simulink model "model"  (R2016a)
settings: Solver=VariableStepAuto  SolverMode=SingleTasking  StartTime=0.0  StopTime=10  RelTol=1e-3
InitFcn:
  | data;
  | ControllerVariant = 'RL';
  | load('rlAgent.mat');
  | doTraining = false;
undefined symbols (not defined in the file): dataType, DiscIntNeverNeededParam, inverter, PI_params, pmsm, PU_System, sigbuilder_block, target, Ts, Ts_motor, Ts_simulink, Ts_speed
libraries: mcbcontrolslib x18, mcbpositiondecoderlib x6, simulink x2, mcbplantlib x1, rllib x1, autolibpmsmexterior x1
settings Model: Creator=Muhammad Umer  LastModifiedBy=Zonularity
settings DataIOCC: ReturnWorkspaceOutputs=on
settings DebuggingCC: ParameterPrecisionLossMsg=none  SFUnexpectedBacktrackingDiag=error  SFNoUnconditionalDefaultTransitionDiag=error
settings SFSimCC: SimUseLocalCustomCode=on
settings RTWCC: RTWUseLocalCustomCode=on
settings GRTTargetCC: TargetLangStandard=C99 (ISO)
settings ConfigComp: CovMetricSettings=dwe  CovSaveCumulativeToWorkspaceVar=off  CovSaveSingleToWorkspaceVar=off  CovExternalEMLEnable=on

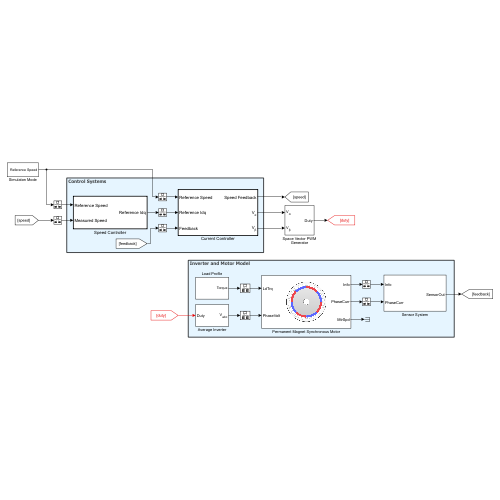
[thumbnail: Simulink's stored preview of the top-level diagram]
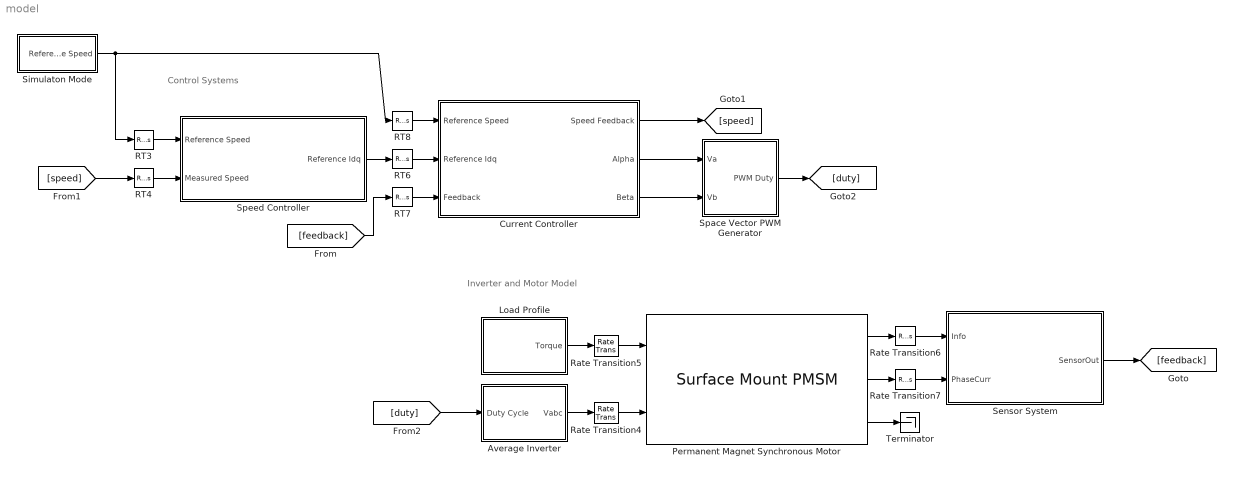
== system model ==
  note: Control Systems
  note: Inverter and Motor Model
  Average Inverter : Subsystem
      mask Display:
      | port_label('input', 1, 'Duty', 'texmode', 'on');
      | port_label('output', 1, 'V_{abc}', 'texmode', 'on');
  Current Controller : Subsystem  TreatAsAtomicUnit=on  mask(Current Controller){contType=PI Controller}
      mask prompts: contType "Controller Type"
      mask help:
      | This block implements the current control loop to generate the desired duty cycle.
      |
      | Choose between a conventional PI Controller and an optimized TD3 Agent.
      mask init:
      | selector = get_param(gcb,'contType');
      | 
      | variantSubsystem = [gcb, '/Control Variant Subsystem']; 
      | 
      | if strcmp(selector,'TD3 Agent')
      |     set_param(variantSubsystem, 'LabelModeActiveChoice', 'RL');
      | else
      |     set_param(variantSubsystem, 'LabelModeActiveChoice', 'PI');
      | end
      settings: OpenFcn=open_system(gcb,'mask');
      mask TypeOptions contType: TD3 Agent | PI Controller
      mask Display:
      | port_label('input', 1, 'Reference Speed', 'texmode', 'on');
      | port_label('input', 2, 'Reference Idq', 'texmode', 'on');
      | port_label('input', 3, 'Feedback', 'texmode', 'on');
      | port_label('output', 1, 'Speed Feedback', 'texmode', 'on');
      | port_label('output', 2, 'V_{\alpha}', 'texmode', 'on');
      | port_label('output', 3, 'V_{\beta}', 'texmode', 'on');
  Load Profile : Subsystem
  Permanent Magnet Synchronous Motor : autolibpmsmexterior/Surface Mount PMSM  port_config=Torque  sim_type=Discrete  Ts=Ts_motor  P=pmsm.p  Rs=pmsm.Rs  Ldq_=pmsm.Ld  KConstText=Permanent flux linkage constant (lambda_pm):  lambda_pm=pmsm.FluxPM  Ke=159.9771  Kt=1.323  mechanical=[pmsm.J, pmsm.B*0, 0]  idq0=[0 0]  theta_init=0  omega_init=0  KConst=pmsm.FluxPM  lambda_pm_calc=pmsm.FluxPM  RefBlkName='autolibpmsmexterior/Surface Mount PMSM'  aMode=5  Ldq="[0.0002      0.0002]"
  RT3 : RateTransition  Deterministic=off  OutPortSampleTime=Ts_speed
  RT4 : RateTransition  Deterministic=off  OutPortSampleTime=Ts_speed
  RT6 : RateTransition  Deterministic=off  OutPortSampleTime=Ts
  RT7 : RateTransition  Deterministic=off  OutPortSampleTime=Ts
  RT8 : RateTransition  Deterministic=off  OutPortSampleTime=Ts
  Rate Transition4 : RateTransition  Deterministic=off  OutPortSampleTime=Ts_motor
  Rate Transition5 : RateTransition  Deterministic=off  OutPortSampleTime=Ts_motor
  Rate Transition6 : RateTransition  Deterministic=off  OutPortSampleTime=Ts_simulink
  Rate Transition7 : RateTransition  Deterministic=off  OutPortSampleTime=Ts_simulink
  Sensor System : Subsystem
      mask Display:
      | port_label('input', 1, 'Info', 'texmode', 'on');
      | port_label('input', 2, 'PhaseCurr', 'texmode', 'on');
      | port_label('output', 1, 'SensorOut', 'texmode', 'on');
  Simulaton Mode : Subsystem  mask(Simulation Mode){Mode=Simulate}
      mask help:
      | Choose simulation mode.
      |
      | Use the training script if the mode is selected to 'Train' Simply run otherwise.
      mask init:
      | selector = get_param(gcb,'Mode');
      | 
      | variantSubsystem = [gcb, '/SimMode']; 
      | 
      | if strcmp(selector,'Simulate')
      |     set_param(variantSubsystem, 'LabelModeActiveChoice', 'simulate');
      | else
      |     set_param(variantSubsystem, 'LabelModeActiveChoice', 'train');
      | end
      settings: OpenFcn=open_system(gcb,'mask');
      mask TypeOptions Mode: Simulate | Train
  Space Vector PWM Generator : Subsystem
      mask Display:
      | color('black');
      | port_label('input', 1, 'V_{\alpha}', 'texmode', 'on');
      | port_label('input', 2, 'V_{\beta}', 'texmode', 'on');
      | port_label('output', 1, 'Duty', 'texmode', 'on');
  Speed Controller : Subsystem  TreatAsAtomicUnit=on  SystemSampleTime=Ts_speed
      mask Display:
      | port_label('input', 1, 'Reference Speed', 'texmode', 'on');
      | port_label('input', 2, 'Measured Speed', 'texmode', 'on');
      | port_label('output', 1, 'Reference Idq', 'texmode', 'on');
  Terminator : Terminator
  wires:
  Rate Transition6/1 -> Sensor System/1(Info)
  Rate Transition4/1 -> Permanent Magnet Synchronous Motor/2
  Rate Transition7/1 -> Sensor System/2(PhaseCurr)
  Load Profile/1(Torque) -> Rate Transition5/1
  Permanent Magnet Synchronous Motor/2 -> Rate Transition7/1
  Average Inverter/1(Vabc) -> Rate Transition4/1
  [speed] -> RT4/1
  Speed Controller/1(Reference Idq) -> RT6/1
  Rate Transition5/1 -> Permanent Magnet Synchronous Motor/1
  Permanent Magnet Synchronous Motor/1 -> Rate Transition6/1
  [feedback] -> RT7/1
  Sensor System/1(SensorOut) -> [feedback]
  Permanent Magnet Synchronous Motor/3 -> Terminator/1
  RT3/1 -> Speed Controller/1(Reference Speed)
  RT4/1 -> Speed Controller/2(Measured Speed)
  [duty] -> Average Inverter/1(Duty Cycle)
  RT8/1 -> Current Controller/1(Reference Speed)
  RT6/1 -> Current Controller/2(Reference Idq)
  RT7/1 -> Current Controller/3(Feedback)
  Current Controller/1(Speed Feedback) -> [speed]
  Simulaton Mode/1(Reference Speed) -> RT3/1, RT8/1
  Current Controller/2(Alpha) -> Space Vector PWM Generator/1(Va)
  Current Controller/3(Beta) -> Space Vector PWM Generator/2(Vb)
  Space Vector PWM Generator/1(PWM Duty) -> [duty]

== system model/Average Inverter ==
  Duty Cycle : Inport
  Average-Value Inverter : mcbplantlib/Average-Value Inverter
  Constant2 : Constant  Value=inverter.V_dc  OutDataTypeStr=single  SampleTime=-1
  Data Type Conversion1 : DataTypeConversion  OutDataTypeStr=single  RndMeth=Simplest
  Rate Transition3 : RateTransition  Integrity=off  Deterministic=off  OutPortSampleTime=Ts_inverter
  Vabc : Outport
  wires:
  Constant2/1 -> Average-Value Inverter/2
  Data Type Conversion1/1 -> Rate Transition3/1
  Rate Transition3/1 -> Average-Value Inverter/1
  Duty Cycle/1 -> Data Type Conversion1/1
  Average-Value Inverter/1 -> Vabc/1

== system model/Current Controller ==
  Reference Speed : Inport
  Reference Idq : Inport  Port=2
  Feedback : Inport  Port=3
  Control Variant Subsystem : Subsystem  Variant=on  OverrideUsingVariant=PI
  Speed Feedback : Outport
  Alpha : Outport  Port=2
  Beta : Outport  Port=3
  wires:
  Control Variant Subsystem/2(Alpha) -> Alpha/1
  Control Variant Subsystem/3(Beta) -> Beta/1
  Control Variant Subsystem/1(Speed Feedback) -> Speed Feedback/1
  Reference Speed/1 -> Control Variant Subsystem/1(Reference Speed)
  Reference Idq/1 -> Control Variant Subsystem/2(Reference Idq)
  Feedback/1 -> Control Variant Subsystem/3(Feedback)

== system model/Load Profile ==
  Data Type Conversion : DataTypeConversion  OutDataTypeStr=single
  Final load : Constant  Value=0.8 * pmsm.T_rated
  IIR Filter : mcbcontrolslib/IIR Filter  VariantControl=Low Pass Filter  VariantSelect=Low-pass  Filter_constant=0.001  advancedSettings=off  Ts=50e-6  cutOff_freq=3.1863
  Motor load : Constant  Commented=on  Value=pmsm.B*pmsm.N_base*2*pi/60
  Switch : Switch  Criteria=u2 > Threshold
  Torque change : Step  Time=19.5  SampleTime=Ts_simulink
  Torque load : Step  Before=0.05*pmsm.T_rated  After=0.5*pmsm.T_rated  SampleTime=Ts_simulink
  Torque : Outport
  wires:
  Switch/1 -> Data Type Conversion/1
  Data Type Conversion/1 -> IIR Filter/1
  Torque change/1 -> Switch/2
  Torque load/1 -> Switch/3
  Final load/1 -> Switch/1
  IIR Filter/1 -> Torque/1

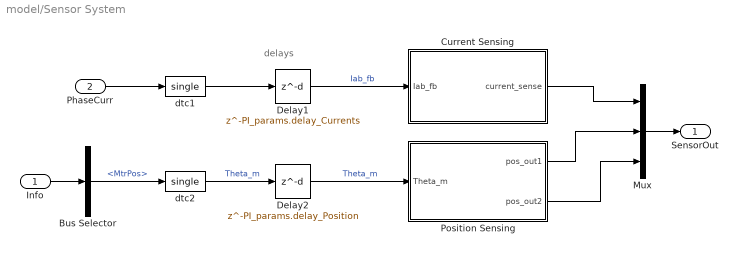
== system model/Sensor System ==
  note: delays
  Info : Inport
  PhaseCurr : Inport  Port=2
  Bus Selector : BusSelector  OutputSignals=MtrPos
  Current Sensing : Subsystem
  Delay1 : Delay  DelayLength=PI_params.delay_Currents
  Delay2 : Delay  DelayLength=PI_params.delay_Position
  Mux : Mux  Inputs=3
  Position Sensing : Subsystem
  dtc1 : DataTypeConversion  OutDataTypeStr=single  RndMeth=Simplest
  dtc2 : DataTypeConversion  OutDataTypeStr=single  RndMeth=Simplest
  SensorOut : Outport
  wires:
  Info/1 -> Bus Selector/1
  PhaseCurr/1 -> dtc1/1
  Bus Selector/1 -> dtc2/1  "<MtrPos>"
  dtc2/1 -> Delay2/1  "Theta_m"
  dtc1/1 -> Delay1/1
  Delay2/1 -> Position Sensing/1(Theta_m)  "Theta_m"
  Delay1/1 -> Current Sensing/1(Iab_fb)  "Iab_fb"
  Current Sensing/1(current_sense) -> Mux/1
  Position Sensing/1(pos_out1) -> Mux/2
  Position Sensing/2(pos_out2) -> Mux/3
  Mux/1 -> SensorOut/1

== system model/Simulaton Mode ==
  SimMode : Subsystem  Variant=on  OverrideUsingVariant=simulate
  Reference Speed : Outport
  wires:
  SimMode/1(Reference Speed) -> Reference Speed/1

== system model/Space Vector PWM Generator ==
  Va : Inport
  Vb : Inport  Port=2
  Mux : Mux  Inputs=3
  Output Scaling : Subsystem
      mask Display:
      | port_label('input', 1, 'V_{abc}', 'texmode', 'on');
      | port_label('output', 1, 'Duty', 'texmode', 'on');
  Space Vector Generator : mcbcontrolslib/Space Vector Generator  inSignal=Valphabeta  modType=SVM: space vector modulation
      link override Modulation method: LabelModeActiveChoice=SVM: space vector modulation
      link override Voltage Input: LabelModeActiveChoice=Valphabeta
  PWM Duty : Outport
  wires:
  Va/1 -> Space Vector Generator/1
  Mux/1 -> Output Scaling/1(Vabc)
  Space Vector Generator/1 -> Mux/1
  Space Vector Generator/3 -> Mux/3
  Space Vector Generator/2 -> Mux/2
  Output Scaling/1(PWM Duty) -> PWM Duty/1
  Vb/1 -> Space Vector Generator/2

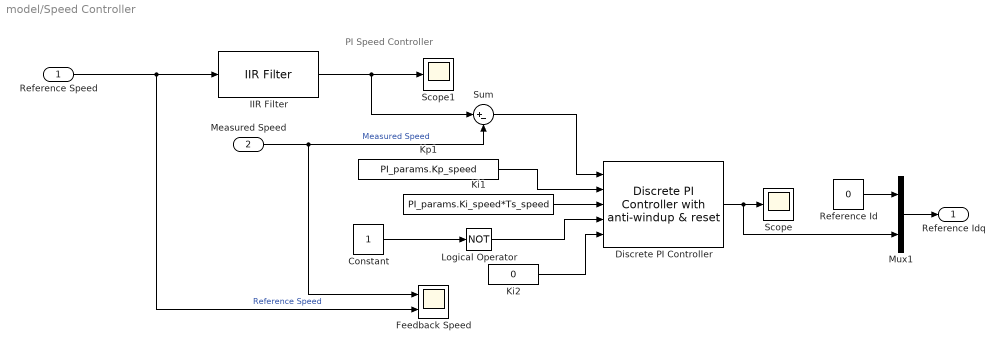
== system model/Speed Controller ==
  note: PI Speed Controller
  Reference Speed : Inport
  Measured Speed : Inport  Port=2
  Constant : Constant  OutDataTypeStr=boolean
  Discrete PI Controller : mcbcontrolslib/Discrete PI Controller  with anti-windup & reset  Controller=PI  UpperSaturationLimit=1  LowerSaturationLimit=-1  IntegratorRTWStateStorageClass=Auto  FilterRTWStateStorageClass=Auto
  Feedback Speed : Scope  NumInputPorts=2
  IIR Filter : mcbcontrolslib/IIR Filter  VariantControl=Low Pass Filter  VariantSelect=Low-pass  Filter_constant=0.01*(Ts_speed/Ts)  advancedSettings=off  Ts=50e-6  cutOff_freq=353.6777
  Ki1 : Constant  Value=PI_params.Ki_speed*Ts_speed  OutDataTypeStr=dataType  SampleTime=-1
  Ki2 : Constant  Value=0  OutDataTypeStr=dataType  SampleTime=-1
  Kp1 : Constant  Value=PI_params.Kp_speed  OutDataTypeStr=dataType  SampleTime=-1
  Logical Operator : Logic  Operator=NOT  IconShape=distinctive  AllPortsSameDT=off  OutDataTypeStr=boolean
  Mux1 : Mux  Inputs=2
  Reference Id : Constant  Value=0  OutDataTypeStr=dataType  SampleTime=Ts_speed
  Scope : Scope
  Scope1 : Scope
  Sum : Sum  Inputs=|+-  OutDataTypeStr=Inherit: Same as first input
  Reference Idq : Outport
  wires:
  Measured Speed/1 -> Feedback Speed/1, Sum/2  "Measured Speed"
  Reference Speed/1 -> Feedback Speed/2, IIR Filter/1  "Reference Speed"
  Reference Id/1 -> Mux1/1
  Mux1/1 -> Reference Idq/1
  IIR Filter/1 -> Sum/1, Scope1/1
  Sum/1 -> Discrete PI Controller/1
  Kp1/1 -> Discrete PI Controller/2
  Ki1/1 -> Discrete PI Controller/3
  Logical Operator/1 -> Discrete PI Controller/4
  Ki2/1 -> Discrete PI Controller/5
  Discrete PI Controller/1 -> Mux1/2, Scope/1
  Constant/1 -> Logical Operator/1

== system model/Current Controller/Control Variant Subsystem ==
  Reference Speed : Inport
  Reference Idq : Inport  Port=2
  Feedback : Inport  Port=3
  PI Controller : Subsystem  VariantControl=PI
  TD3 Agent : Subsystem  VariantControl=RL
  Speed Feedback : Outport
  Alpha : Outport  Port=2
  Beta : Outport  Port=3

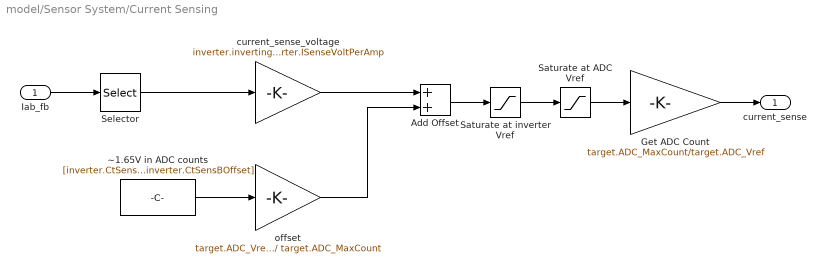
== system model/Sensor System/Current Sensing ==
  Iab_fb : Inport
  Add Offset : Sum  RndMeth=Simplest
  Get ADC Count : Gain  Gain=target.ADC_MaxCount/target.ADC_Vref  OutMin=0  OutMax=target.ADC_MaxCount  OutDataTypeStr=uint16  RndMeth=Simplest
  Saturate at ADC Vref : Saturate  UpperLimit=target.ADC_Vref  LowerLimit=0
  Saturate at inverter Vref : Saturate  UpperLimit=inverter.ISenseVref  LowerLimit=0
  Selector : Selector  InputPortWidth=3  IndexOptions=Index vector (dialog)  Indices=[1 2]  OutputSizes=1
  current_sense_voltage : Gain  Gain=inverter.invertingAmp * inverter.ISenseVoltPerAmp  RndMeth=Simplest  OutDataTypeStr=Inherit: Same as input
  offset : Gain  Gain=target.ADC_Vref / target.ADC_MaxCount  RndMeth=Simplest
  ~1.65V in ADC counts : Constant  Value=[inverter.CtSensAOffset inverter.CtSensBOffset]  OutDataTypeStr=uint16  SampleTime=-1
  current_sense : Outport
  wires:
  Iab_fb/1 -> Selector/1
  current_sense_voltage/1 -> Add Offset/1
  Get ADC Count/1 -> current_sense/1
  ~1.65V in ADC counts/1 -> offset/1
  offset/1 -> Add Offset/2
  Saturate at ADC Vref/1 -> Get ADC Count/1
  Selector/1 -> current_sense_voltage/1
  Saturate at inverter Vref/1 -> Saturate at ADC Vref/1
  Add Offset/1 -> Saturate at inverter Vref/1

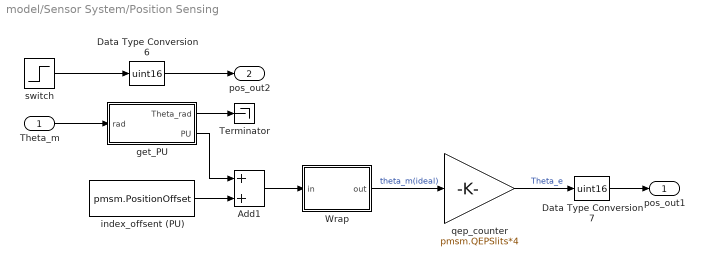
== system model/Sensor System/Position Sensing ==
  Theta_m : Inport
  Add1 : Sum  RndMeth=Simplest
  Data Type Conversion6 : DataTypeConversion  OutDataTypeStr=uint16  RndMeth=Simplest
  Data Type Conversion7 : DataTypeConversion  OutDataTypeStr=uint16  RndMeth=Simplest
  Terminator : Terminator
  Wrap : Subsystem
  "get_PU " : Subsystem
  index_offsent (PU) : Constant  Value=pmsm.PositionOffset  OutDataTypeStr=single  SampleTime=-1
  qep_counter : Gain  Gain=pmsm.QEPSlits*4  OutDataTypeStr=uint16  RndMeth=Simplest
  switch : Step  Time=0.1  SampleTime=Ts_motor
  pos_out1 : Outport
  pos_out2 : Outport  Port=2
  wires:
  Add1/1 -> Wrap/1(in)
  index_offsent (PU)/1 -> Add1/2
  qep_counter/1 -> Data Type Conversion7/1  "Theta_e"
  Theta_m/1 -> "get_PU "/1(rad)
  Data Type Conversion7/1 -> pos_out1/1
  Data Type Conversion6/1 -> pos_out2/1
  switch/1 -> Data Type Conversion6/1
  Wrap/1(out) -> qep_counter/1  "theta_m(ideal)"
  "get_PU "/2(PU) -> Add1/1
  "get_PU "/1(Theta_rad) -> Terminator/1

== system model/Simulaton Mode/SimMode ==
  Simulator : Subsystem  VariantControl=simulate
  Trainer : Subsystem  VariantControl=train
  Reference Speed : Outport

== system model/Space Vector PWM Generator/Output Scaling ==
  Vabc : Inport
  Constant : Constant  Value=0.5  OutDataTypeStr=dataType
  Gain : Gain  Gain=0.5  OutDataTypeStr=dataType  RndMeth=Simplest
  Sum : Sum  Inputs=|++
  PWM Duty : Outport
  wires:
  Sum/1 -> PWM Duty/1  "Duty Cycles"
  Vabc/1 -> Gain/1
  Gain/1 -> Sum/1
  Constant/1 -> Sum/2

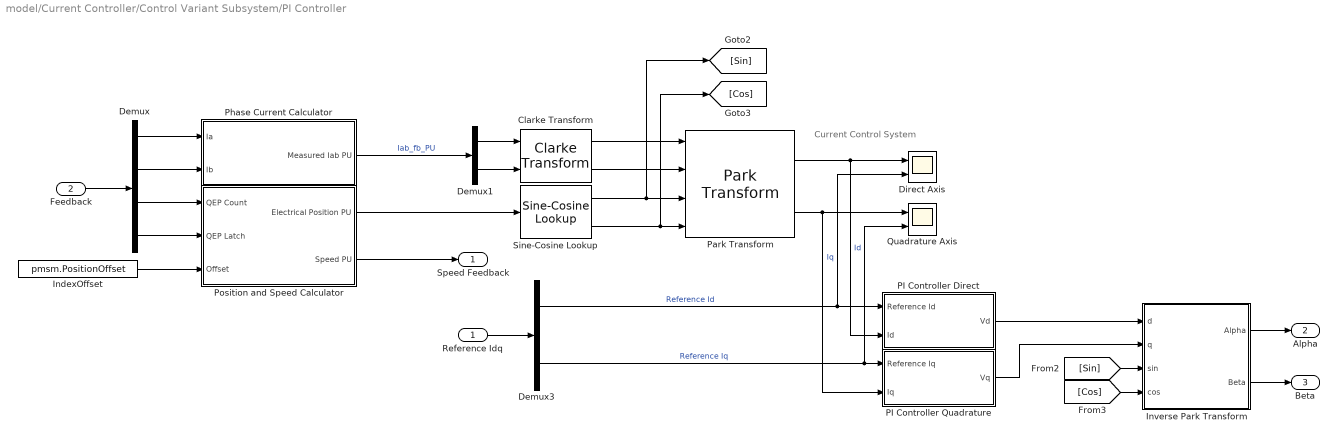
== system model/Current Controller/Control Variant Subsystem/PI Controller ==
  note: Current Control System
  Reference Idq : Inport
  Feedback : Inport  Port=2
  Clarke Transform : mcbcontrolslib/Clarke Transform  VariantControl=Variant2
  Demux : Demux
  Demux1 : Demux  Outputs=2
  Demux3 : Demux  Outputs=2
  Direct Axis : Scope  NumInputPorts=2
  IndexOffset : Constant  Value=pmsm.PositionOffset  OutDataTypeStr=dataType  SampleTime=-1
  Inverse Park Transform : Subsystem
      mask Display:
      | port_label('output', 1, 'V_{\alpha}', 'texmode', 'on');
      | port_label('output', 2, 'V_{\beta}', 'texmode', 'on');
      | port_label('input', 1, 'd', 'texmode', 'on');
      | port_label('input', 2, 'q', 'texmode', 'on');
      | port_label('input', 3, 'sin\theta_{e}', 'texmode', 'on');
      | port_label('input', 4, 'cos\theta_{e}', 'texmode', 'on');
  PI Controller Direct : Subsystem
  PI Controller Quadrature : Subsystem
  Park Transform : mcbcontrolslib/Park Transform  AxisAlignment=D-axis
  Phase Current Calculator : Subsystem
  Position and Speed Calculator : Subsystem
  Quadrature Axis : Scope  NumInputPorts=2
  Sine-Cosine Lookup : mcbcontrolslib/Sine-Cosine Lookup  AngleInput=Per-unit  N_points=1024
  Speed Feedback : Outport  InitialOutput=0
  Alpha : Outport  Port=2
  Beta : Outport  Port=3
  wires:
  Clarke Transform/1 -> Park Transform/1
  Inverse Park Transform/1(Alpha) -> Alpha/1
  Clarke Transform/2 -> Park Transform/2
  Sine-Cosine Lookup/2 -> [Cos], Park Transform/4
  [Sin] -> Inverse Park Transform/3(sin)
  Feedback/1 -> Demux/1
  Demux/2 -> Phase Current Calculator/2(Ib)
  Demux3/1 -> Direct Axis/2, PI Controller Direct/1(Reference Id)  "Reference Id"
  Demux1/1 -> Clarke Transform/1
  Position and Speed Calculator/1(Electrical Position PU) -> Sine-Cosine Lookup/1
  IndexOffset/1 -> Position and Speed Calculator/3(Offset)
  Demux/1 -> Phase Current Calculator/1(Ia)
  Position and Speed Calculator/2(Speed PU) -> Speed Feedback/1
  [Cos] -> Inverse Park Transform/4(cos)
  Inverse Park Transform/2(Beta) -> Beta/1
  Sine-Cosine Lookup/1 -> [Sin], Park Transform/3
  Demux1/2 -> Clarke Transform/2
  Reference Idq/1 -> Demux3/1
  Demux/3 -> Position and Speed Calculator/1(QEP Count)
  Demux/4 -> Position and Speed Calculator/2(QEP Latch)
  Phase Current Calculator/1(Measured Iab PU) -> Demux1/1  "Iab_fb_PU"
  Demux3/2 -> Quadrature Axis/2, PI Controller Quadrature/1(Reference Iq)  "Reference Iq"
  Park Transform/1 -> Direct Axis/1, PI Controller Direct/2(Id)  "Id"
  Park Transform/2 -> Quadrature Axis/1, PI Controller Quadrature/2(Iq)  "Iq"
  PI Controller Direct/1(Vd) -> Inverse Park Transform/1(d)
  PI Controller Quadrature/1(Vq) -> Inverse Park Transform/2(q)

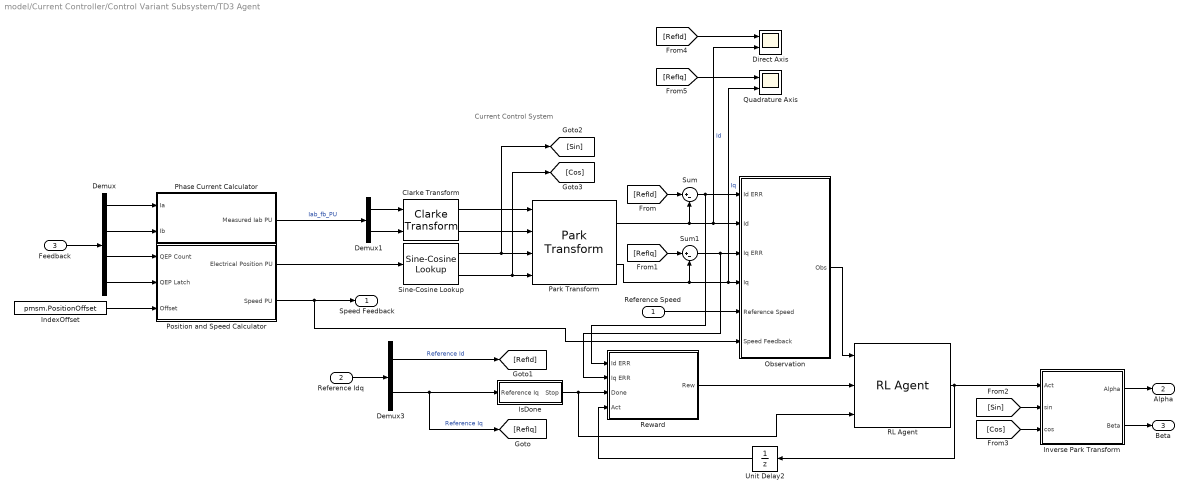
== system model/Current Controller/Control Variant Subsystem/TD3 Agent ==
  note: Current Control System
  Reference Speed : Inport
  Reference Idq : Inport  Port=2
  Feedback : Inport  Port=3
  Clarke Transform : mcbcontrolslib/Clarke Transform  VariantControl=Variant2
  Demux : Demux
  Demux1 : Demux  Outputs=2
  Demux3 : Demux  Outputs=2
  Direct Axis : Scope  NumInputPorts=2
  IndexOffset : Constant  Value=pmsm.PositionOffset  OutDataTypeStr=dataType  SampleTime=-1
  Inverse Park Transform : Subsystem
      mask Display:
      | port_label('output', 1, 'V_{\alpha}', 'texmode', 'on');
      | port_label('output', 2, 'V_{\beta}', 'texmode', 'on');
      | port_label('input', 1, 'Act', 'texmode', 'on');
      | port_label('input', 2, 'sin\theta_{e}', 'texmode', 'on');
      | port_label('input', 3, 'cos\theta_{e}', 'texmode', 'on');
  IsDone : Subsystem
  Observation : Subsystem
  Park Transform : mcbcontrolslib/Park Transform  AxisAlignment=D-axis
  Phase Current Calculator : Subsystem
  Position and Speed Calculator : Subsystem
  Quadrature Axis : Scope  NumInputPorts=2
  RL Agent : rllib/RL Agent  Agent=agent  ExternalActionAsInput=off  ProvideLastAction=off  ProvideCumRwd=off  TreatAsDirectFeedthrough=on  UseStrictObservationDataTypes=off
  Reward : Subsystem
  Sine-Cosine Lookup : mcbcontrolslib/Sine-Cosine Lookup  AngleInput=Per-unit  N_points=1024
  Sum : Sum  Inputs=|+-  OutDataTypeStr=Inherit: Inherit via back propagation
  Sum1 : Sum  Inputs=|+-  OutDataTypeStr=Inherit: Inherit via back propagation
  Unit Delay2 : UnitDelay  SampleTime=-1  HasFrameUpgradeWarning=on
  Speed Feedback : Outport  InitialOutput=0
  Alpha : Outport  Port=2
  Beta : Outport  Port=3
  wires:
  IndexOffset/1 -> Position and Speed Calculator/3(Offset)
  Sum1/1 -> Reward/2(Iq ERR), Observation/3(Iq ERR)
  Reward/1(Rew) -> RL Agent/2
  Sum/1 -> Reward/1(Id ERR), Observation/1(Id ERR)
  Demux/1 -> Phase Current Calculator/1(Ia)
  Demux/3 -> Position and Speed Calculator/1(QEP Count)
  [RefIq] -> Sum1/1
  Park Transform/2 -> Sum1/2, Quadrature Axis/2, Observation/4(Iq)  "Iq"
  Inverse Park Transform/2(Beta) -> Beta/1
  Demux1/2 -> Clarke Transform/2
  IsDone/1(Stop) -> RL Agent/3, Reward/3(Done)
  Observation/1(Obs) -> RL Agent/1
  Inverse Park Transform/1(Alpha) -> Alpha/1
  [Cos] -> Inverse Park Transform/3(cos)
  Feedback/1 -> Demux/1
  Demux3/1 -> [RefId]  "Reference Id"
  Demux/2 -> Phase Current Calculator/2(Ib)
  Sine-Cosine Lookup/1 -> [Sin], Park Transform/3
  Park Transform/1 -> Sum/2, Direct Axis/2, Observation/2(Id)  "Id"
  Position and Speed Calculator/2(Speed PU) -> Observation/6(Speed Feedback), Speed Feedback/1
  Demux3/2 -> [RefIq], IsDone/1(Reference Iq)  "Reference Iq"
  Demux/4 -> Position and Speed Calculator/2(QEP Latch)
  Demux1/1 -> Clarke Transform/1
  [Sin] -> Inverse Park Transform/2(sin)
  Sine-Cosine Lookup/2 -> [Cos], Park Transform/4
  Reference Speed/1 -> Observation/5(Reference Speed)
  Position and Speed Calculator/1(Electrical Position PU) -> Sine-Cosine Lookup/1
  Reference Idq/1 -> Demux3/1
  Unit Delay2/1 -> Reward/4(Act)
  Clarke Transform/1 -> Park Transform/1
  Phase Current Calculator/1(Measured Iab PU) -> Demux1/1  "Iab_fb_PU"
  RL Agent/1 -> Inverse Park Transform/1(Act), Unit Delay2/1
  [RefId] -> Sum/1
  Clarke Transform/2 -> Park Transform/2
  [RefIq] -> Quadrature Axis/1
  [RefId] -> Direct Axis/1

== system model/Sensor System/Position Sensing/Wrap ==
  in : Inport
  Constant2 : Constant  OutDataTypeStr=single  SampleTime=-1
  Mod : Math  Operator=mod  SaturateOnIntegerOverflow=on
  out : Outport
  wires:
  in/1 -> Mod/1
  Constant2/1 -> Mod/2
  Mod/1 -> out/1

== system model/Sensor System/Position Sensing/get_PU  ==
  rad : Inport
  Constant2 : Constant  Value=2*pi  OutDataTypeStr=single  SampleTime=-1
  Get_PU : Gain  Gain=1/(2*pi)  RndMeth=Simplest  OutDataTypeStr=Inherit: Same as input
  Mod : Math  Operator=mod  SaturateOnIntegerOverflow=on
  Theta_rad : Outport
  PU : Outport  Port=2
  wires:
  rad/1 -> Mod/1
  Constant2/1 -> Mod/2
  Mod/1 -> Theta_rad/1, Get_PU/1
  Get_PU/1 -> PU/1

== system model/Simulaton Mode/SimMode/Simulator ==
  Signal Builder : Subsystem  Tag=STV Subsys  LoadFcn=sigbuilder_block('load');  StartFcn=sigbuilder_block('start');  StopFcn=sigbuilder_block('stop');  ClipboardFcn=sigbuilder_block('clipboard');  mask(Sigbuilder block){}
      mask help: Simulink:masks:SigbuilderBlock_MD
      mask init:
      | if ~strcmp(get_param(bdroot(gcbh),'SimulationStatus'),'stopped') tuvar = sigbuilder_block('maskInit'); end
      settings: CopyFcn=sigbuilder_block('copy');  DeleteFcn=sigbuilder_block('delete');  ModelCloseFcn=sigbuilder_block('modelClose');  PreSaveFcn=sigbuilder_block('preSave');  PauseFcn=sigbuilder_block('pause');  ContinueFcn=sigbuilder_block('continue');  NameChangeFcn=sigbuilder_block('namechange');  OpenFcn=sigbuilder_block('open',[437.25 199.5 550.5 399.75 ]);  CloseFcn=sigbuilder_block('close');
      mask Display: plot(0, 0, 100, 100,[2, 2, 32, 32, 2], [68, 8, 8, 68, 68],[32, 2], [38, 38], [32, 19, 2],[53, 60, 44], [32, 17, 17, 2],[16, 16, 31, 31]);txt = getActiveGroup(gcbh);text(2, 100, txt,'verticalAlignment', 'top');
  dtc : DataTypeConversion  OutDataTypeStr=dataType
  Reference Speed : Outport
  wires:
  dtc/1 -> Reference Speed/1
  Signal Builder/1(PU) -> dtc/1

== system model/Simulaton Mode/SimMode/Trainer ==
  Data Type Conversion : DataTypeConversion  OutDataTypeStr=dataType
  SpeedRef : Step  Time=0  After=0.6  SampleTime=Ts_speed
  Reference Speed : Outport
  wires:
  SpeedRef/1 -> Data Type Conversion/1
  Data Type Conversion/1 -> Reference Speed/1

== system model/Current Controller/Control Variant Subsystem/PI Controller/Inverse Park Transform ==
  d : Inport
  q : Inport  Port=2
  sin : Inport  Port=3
  cos : Inport  Port=4
  DQ Limiter : mcbcontrolslib/DQ Limiter  Vmax=0.95
  Inverse Park Transform : mcbcontrolslib/Inverse Park Transform  AxisAlignment=D-axis
  Terminator : Terminator
  Alpha : Outport
  Beta : Outport  Port=2
  wires:
  DQ Limiter/2 -> Inverse Park Transform/2  "Vq"
  DQ Limiter/1 -> Inverse Park Transform/1  "Vd"
  sin/1 -> Inverse Park Transform/3
  Inverse Park Transform/1 -> Alpha/1
  DQ Limiter/3 -> Terminator/1
  d/1 -> DQ Limiter/1
  cos/1 -> Inverse Park Transform/4
  Inverse Park Transform/2 -> Beta/1
  q/1 -> DQ Limiter/2

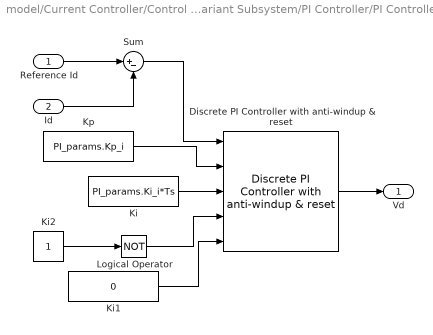
== system model/Current Controller/Control Variant Subsystem/PI Controller/PI Controller Direct ==
  Reference Id : Inport
  Id : Inport  Port=2
  Discrete PI Controller with anti-windup & reset : mcbcontrolslib/Discrete PI Controller  with anti-windup & reset  Controller=PI  UpperSaturationLimit=1  LowerSaturationLimit=-1  IntegratorRTWStateStorageClass=Auto  FilterRTWStateStorageClass=Auto
  Ki : Constant  Value=PI_params.Ki_i*Ts  OutDataTypeStr=dataType  SampleTime=-1
  Ki1 : Constant  Value=0  OutDataTypeStr=dataType  SampleTime=-1
  Ki2 : Constant  OutDataTypeStr=boolean  SampleTime=-1
  Kp : Constant  Value=PI_params.Kp_i  OutDataTypeStr=dataType  SampleTime=-1
  Logical Operator : Logic  Operator=NOT  IconShape=distinctive  AllPortsSameDT=off  OutDataTypeStr=boolean
  Sum : Sum  Inputs=|+-  OutDataTypeStr=Inherit: Same as first input
  Vd : Outport
  wires:
  Ki2/1 -> Logical Operator/1
  Sum/1 -> Discrete PI Controller with anti-windup & reset/1
  Ki1/1 -> Discrete PI Controller with anti-windup & reset/5
  Id/1 -> Sum/2
  Kp/1 -> Discrete PI Controller with anti-windup & reset/2
  Logical Operator/1 -> Discrete PI Controller with anti-windup & reset/4
  Discrete PI Controller with anti-windup & reset/1 -> Vd/1
  Ki/1 -> Discrete PI Controller with anti-windup & reset/3
  Reference Id/1 -> Sum/1

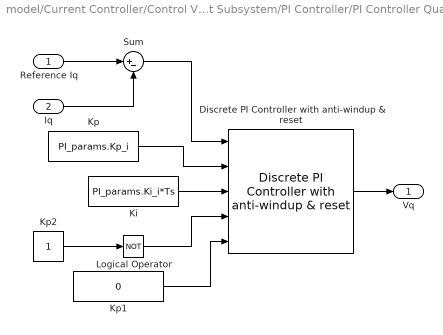
== system model/Current Controller/Control Variant Subsystem/PI Controller/PI Controller Quadrature ==
  Reference Iq : Inport
  Iq : Inport  Port=2
  Discrete PI Controller with anti-windup & reset : mcbcontrolslib/Discrete PI Controller  with anti-windup & reset  Controller=PI  UpperSaturationLimit=1  LowerSaturationLimit=-1  IntegratorRTWStateStorageClass=Auto  FilterRTWStateStorageClass=Auto
  Ki : Constant  Value=PI_params.Ki_i*Ts  OutDataTypeStr=dataType  SampleTime=-1
  Kp : Constant  Value=PI_params.Kp_i  OutDataTypeStr=dataType  SampleTime=-1
  Kp1 : Constant  Value=0  OutDataTypeStr=dataType  SampleTime=-1
  Kp2 : Constant  OutDataTypeStr=boolean  SampleTime=-1
  Logical Operator : Logic  Operator=NOT  IconShape=distinctive  AllPortsSameDT=off  OutDataTypeStr=boolean
  Sum : Sum  Inputs=|+-  OutDataTypeStr=Inherit: Same as first input
  Vq : Outport
  wires:
  Ki/1 -> Discrete PI Controller with anti-windup & reset/3
  Sum/1 -> Discrete PI Controller with anti-windup & reset/1
  Kp1/1 -> Discrete PI Controller with anti-windup & reset/5
  Kp2/1 -> Logical Operator/1
  Kp/1 -> Discrete PI Controller with anti-windup & reset/2
  Logical Operator/1 -> Discrete PI Controller with anti-windup & reset/4
  Reference Iq/1 -> Sum/1
  Iq/1 -> Sum/2
  Discrete PI Controller with anti-windup & reset/1 -> Vq/1

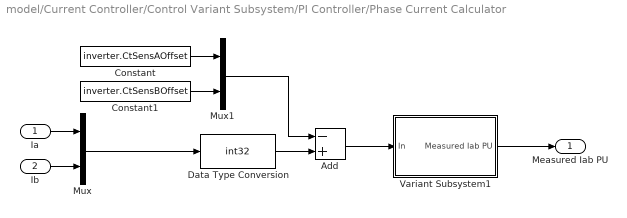
== system model/Current Controller/Control Variant Subsystem/PI Controller/Phase Current Calculator ==
  Ia : Inport
  Ib : Inport  Port=2
  Add : Sum  Inputs=-+
  Constant : Constant  Value=inverter.CtSensAOffset  OutDataTypeStr=uint16
  Constant1 : Constant  Value=inverter.CtSensBOffset  OutDataTypeStr=uint16
  Data Type Conversion : DataTypeConversion  OutDataTypeStr=int32  ConvertRealWorld=Stored Integer (SI)  RndMeth=Simplest
  Mux : Mux  Inputs=2
  Mux1 : Mux  Inputs=2
  Variant Subsystem1 : Subsystem  Variant=on
  Measured Iab PU : Outport
  wires:
  Variant Subsystem1/1(Measured Iab PU) -> Measured Iab PU/1
  Add/1 -> Variant Subsystem1/1(In)
  Data Type Conversion/1 -> Add/2
  Ib/1 -> Mux/2
  Constant/1 -> Mux1/1
  Ia/1 -> Mux/1
  Constant1/1 -> Mux1/2
  Mux/1 -> Data Type Conversion/1
  Mux1/1 -> Add/1

== system model/Current Controller/Control Variant Subsystem/PI Controller/Position and Speed Calculator ==
  QEP Count : Inport
  QEP Latch : Inport  Port=2
  Offset : Inport  Port=3
  IIR Filter : mcbcontrolslib/IIR Filter  VariantControl=Low Pass Filter  VariantSelect=Low-pass  Filter_constant=0.01  advancedSettings=off  Ts=50e-6  cutOff_freq=32.1525
  Mechanical to Electrical Position : mcbpositiondecoderlib/Mechanical to Electrical Position  NrPP=pmsm.p  selectedRange=Per unit  MechOfstInputType=Input port  mechOffsetIn=0  maxAngleIn=1  InputDataType=dataType  VariantSelect=floating-point
  Quadrature Decoder : mcbpositiondecoderlib/Quadrature Decoder  EncoderSlitsPerRevolution=pmsm.QEPSlits  EncoderCountsPerSlit=4  CounterSize=16 bits  ExternalIndexCount=on  PositionUnit=Per unit  PositionDataType=dataType
  Speed Measurement : mcbpositiondecoderlib/Speed Measurement  PositionUnit=Per unit  PositionScalingDatatype=uint32  SpeedCalculationMode=Time interval for speed calculation  SampleTimeAsync=Ts  MaximumApplicationSpeed=6000  SpeedResolution=5e-6  DelayLength=20  MaximumMeasurableSpeed=7499  MeasurableSpeedResolution=3.4925e-06  SpeedUnit=Per unit based on dialog  PerUnitSpeed=PU_System.N_base  SpeedDataType=dataType
  Electrical Position PU : Outport
  Speed PU : Outport  Port=2
  wires:
  Quadrature Decoder/1 -> Mechanical to Electrical Position/1, Speed Measurement/1
  Mechanical to Electrical Position/1 -> Electrical Position PU/1
  Speed Measurement/1 -> IIR Filter/1
  QEP Latch/1 -> Quadrature Decoder/2
  IIR Filter/1 -> Speed PU/1
  Offset/1 -> Mechanical to Electrical Position/2
  QEP Count/1 -> Quadrature Decoder/1

== system model/Current Controller/Control Variant Subsystem/TD3 Agent/Inverse Park Transform ==
  Act : Inport
  sin : Inport  Port=2
  cos : Inport  Port=3
  DQ Limiter : mcbcontrolslib/DQ Limiter  Vmax=0.95
  Data Type Conversion : DataTypeConversion  OutDataTypeStr=dataType
  Demux2 : Demux  Outputs=2
  Inverse Park Transform : mcbcontrolslib/Inverse Park Transform  AxisAlignment=D-axis
  Terminator : Terminator
  Alpha : Outport
  Beta : Outport  Port=2
  wires:
  DQ Limiter/2 -> Inverse Park Transform/2  "Vq"
  DQ Limiter/1 -> Inverse Park Transform/1  "Vd"
  sin/1 -> Inverse Park Transform/3
  Demux2/2 -> DQ Limiter/2
  Inverse Park Transform/1 -> Alpha/1
  DQ Limiter/3 -> Terminator/1
  Act/1 -> Data Type Conversion/1
  Demux2/1 -> DQ Limiter/1
  Data Type Conversion/1 -> Demux2/1
  cos/1 -> Inverse Park Transform/4
  Inverse Park Transform/2 -> Beta/1

== system model/Current Controller/Control Variant Subsystem/TD3 Agent/IsDone ==
  Reference Iq : Inport
  Compare To Constant2 : simulink/Logic and Bit Operations/Compare To Constant  relop=>=  const=0.3  OutDataTypeStr=boolean
  Compare To Constant3 : simulink/Logic and Bit Operations/Compare To Constant  relop=>=  const=1  OutDataTypeStr=boolean
  Digital Clock : DigitalClock  SampleTime=Ts
  OR1 : Logic  IconShape=distinctive  AllPortsSameDT=off  OutDataTypeStr=boolean
  Product : Product
  Trainer : Constant  OutDataTypeStr=double
  Stop : Outport
  wires:
  Trainer/1 -> Product/2
  Product/1 -> Stop/1
  Digital Clock/1 -> Compare To Constant2/1
  OR1/1 -> Product/1
  Compare To Constant3/1 -> OR1/1
  Reference Iq/1 -> Compare To Constant3/1
  Compare To Constant2/1 -> OR1/2

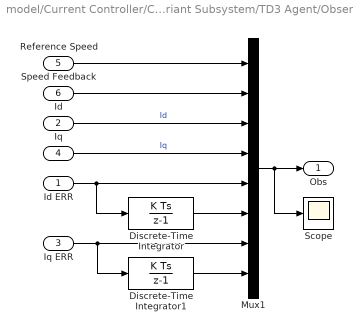
== system model/Current Controller/Control Variant Subsystem/TD3 Agent/Observation ==
  Id ERR : Inport
  Id : Inport  Port=2
  Iq ERR : Inport  Port=3
  Iq : Inport  Port=4
  Reference Speed : Inport  Port=5
  Speed Feedback : Inport  Port=6
  Discrete-Time Integrator : DiscreteIntegrator  InitialConditionSetting=State (most efficient)  SampleTime=-1  LimitOutput=on  UpperSaturationLimit=0.05  LowerSaturationLimit=0  ICPrevOutput=DiscIntNeverNeededParam  ICPrevScaledInput=DiscIntNeverNeededParam
  Discrete-Time Integrator1 : DiscreteIntegrator  InitialConditionSetting=State (most efficient)  SampleTime=-1  LimitOutput=on  UpperSaturationLimit=0.05  LowerSaturationLimit=0  ICPrevOutput=DiscIntNeverNeededParam  ICPrevScaledInput=DiscIntNeverNeededParam
  Mux1 : Mux  Inputs=8
  Scope : Scope
  Obs : Outport
  wires:
  Id ERR/1 -> Discrete-Time Integrator/1, Mux1/5
  Discrete-Time Integrator/1 -> Mux1/6
  Iq ERR/1 -> Discrete-Time Integrator1/1, Mux1/7
  Discrete-Time Integrator1/1 -> Mux1/8
  Mux1/1 -> Obs/1, Scope/1
  Iq/1 -> Mux1/4  "Iq"
  Id/1 -> Mux1/3  "Id"
  Speed Feedback/1 -> Mux1/2
  Reference Speed/1 -> Mux1/1

== system model/Current Controller/Control Variant Subsystem/TD3 Agent/Phase Current Calculator ==
  Ia : Inport
  Ib : Inport  Port=2
  Add : Sum  Inputs=-+
  Constant : Constant  Value=inverter.CtSensAOffset  OutDataTypeStr=uint16
  Constant1 : Constant  Value=inverter.CtSensBOffset  OutDataTypeStr=uint16
  Data Type Conversion : DataTypeConversion  OutDataTypeStr=int32  ConvertRealWorld=Stored Integer (SI)  RndMeth=Simplest
  Mux : Mux  Inputs=2
  Mux1 : Mux  Inputs=2
  Variant Subsystem1 : Subsystem  Variant=on
  Measured Iab PU : Outport
  wires:
  Variant Subsystem1/1(Measured Iab PU) -> Measured Iab PU/1
  Add/1 -> Variant Subsystem1/1(In)
  Data Type Conversion/1 -> Add/2
  Ib/1 -> Mux/2
  Constant/1 -> Mux1/1
  Ia/1 -> Mux/1
  Constant1/1 -> Mux1/2
  Mux/1 -> Data Type Conversion/1
  Mux1/1 -> Add/1

== system model/Current Controller/Control Variant Subsystem/TD3 Agent/Position and Speed Calculator ==
  QEP Count : Inport
  QEP Latch : Inport  Port=2
  Offset : Inport  Port=3
  IIR Filter : mcbcontrolslib/IIR Filter  VariantControl=Low Pass Filter  VariantSelect=Low-pass  Filter_constant=0.01  advancedSettings=off  Ts=50e-6  cutOff_freq=32.1525
  Mechanical to Electrical Position : mcbpositiondecoderlib/Mechanical to Electrical Position  NrPP=pmsm.p  selectedRange=Per unit  MechOfstInputType=Input port  mechOffsetIn=0  maxAngleIn=1  InputDataType=dataType  VariantSelect=floating-point
  Quadrature Decoder : mcbpositiondecoderlib/Quadrature Decoder  EncoderSlitsPerRevolution=pmsm.QEPSlits  EncoderCountsPerSlit=4  CounterSize=16 bits  ExternalIndexCount=on  PositionUnit=Per unit  PositionDataType=dataType
  Speed Measurement : mcbpositiondecoderlib/Speed Measurement  PositionUnit=Per unit  PositionScalingDatatype=uint32  SpeedCalculationMode=Time interval for speed calculation  SampleTimeAsync=Ts  MaximumApplicationSpeed=6000  SpeedResolution=5e-6  DelayLength=20  MaximumMeasurableSpeed=7499  MeasurableSpeedResolution=3.4925e-06  SpeedUnit=Per unit based on dialog  PerUnitSpeed=PU_System.N_base  SpeedDataType=dataType
  Electrical Position PU : Outport
  Speed PU : Outport  Port=2
  wires:
  Quadrature Decoder/1 -> Mechanical to Electrical Position/1, Speed Measurement/1
  Mechanical to Electrical Position/1 -> Electrical Position PU/1
  Speed Measurement/1 -> IIR Filter/1
  QEP Latch/1 -> Quadrature Decoder/2
  IIR Filter/1 -> Speed PU/1
  Offset/1 -> Mechanical to Electrical Position/2
  QEP Count/1 -> Quadrature Decoder/1

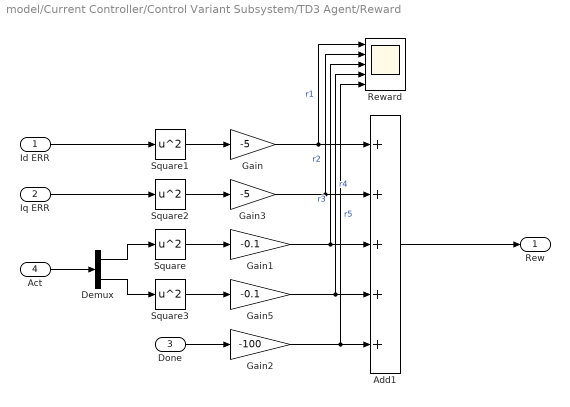
== system model/Current Controller/Control Variant Subsystem/TD3 Agent/Reward ==
  Id ERR : Inport
  Iq ERR : Inport  Port=2
  Done : Inport  Port=3
  Act : Inport  Port=4
  Add1 : Sum  Inputs=+++++
  Demux : Demux  Outputs=2
  Gain : Gain  Gain=-5
  Gain1 : Gain  Gain=-0.1
  Gain2 : Gain  Gain=-100
  Gain3 : Gain  Gain=-5
  Gain5 : Gain  Gain=-0.1
  Reward : Scope  NumInputPorts=5
  Square{,1..3} (4 alike) : Math  Operator=square  SaturateOnIntegerOverflow=on
  Rew : Outport
  wires:
  Done/1 -> Gain2/1
  Gain2/1 -> Reward/5, Add1/5  "r5"
  Iq ERR/1 -> Square2/1
  Id ERR/1 -> Square1/1
  Gain3/1 -> Add1/2, Reward/2  "r2"
  Gain/1 -> Add1/1, Reward/1  "r1"
  Gain5/1 -> Add1/4, Reward/4  "r4"
  Add1/1 -> Rew/1
  Act/1 -> Demux/1
  Square3/1 -> Gain5/1
  Demux/2 -> Square3/1
  Gain1/1 -> Add1/3, Reward/3  "r3"
  Square/1 -> Gain1/1
  Demux/1 -> Square/1
  Square2/1 -> Gain3/1
  Square1/1 -> Gain/1

== system model/Simulaton Mode/SimMode/Simulator/Signal Builder ==
  Demux : Demux  Tag=STV Demux  Outputs=1
      settings: DisplayOption=none
  FromWs : FromWorkspace  Tag=STV FromWs  VariableName=tuvar
      SigBuilderData=|
      | common.afterFinalStr = 'Extrapolate'
      | common.sampleTime = 0
      | dataSet.timeRange = [0 10]
      | dataSet.name = 'Reference Speed'
      | sbobj.Groups.Name = 'Reference Speed'
      | sbobj.Groups.Signals.Name = 'PU'
      | sbobj.Groups.Signals.XData = [0 1 1 2 2 3 4 4 5 5 6 6 7 7 8 8 9 9 10]
      | sbobj.Groups.Signals.YData = [0.2 0.2 0.4 0.4 0.6 0.6 0.6 0.2 0.2 0.8 0.8 0.4 0.4 0.8 0.8 0.6 0.6 0.4 0.4]
  PU : Outport  Tag=STV Outport
  wires:
  FromWs/1 -> Demux/1
  Demux/1 -> PU/1

== system model/Current Controller/Control Variant Subsystem/PI Controller/Phase Current Calculator/Variant Subsystem1 ==
  In : Inport
  Fixed Point : Subsystem  VariantControl=~isequal(dataType,'single')
  Float : Subsystem  VariantControl=isequal(dataType,'single')
  Measured Iab PU : Outport

== system model/Current Controller/Control Variant Subsystem/TD3 Agent/Phase Current Calculator/Variant Subsystem1 ==
  In : Inport
  Fixed Point : Subsystem  VariantControl=~isequal(dataType,'single')
  Float : Subsystem  VariantControl=isequal(dataType,'single')
  Measured Iab PU : Outport

== system model/Current Controller/Control Variant Subsystem/PI Controller/Phase Current Calculator/Variant Subsystem1/Fixed Point ==
  In : Inport
  Data Type Conversion : DataTypeConversion  OutDataTypeStr=fixdt(1,32,17)  ConvertRealWorld=Stored Integer (SI)  RndMeth=Simplest
  Data Type Conversion1 : DataTypeConversion  OutDataTypeStr=dataType  RndMeth=Simplest
  Q17 per unit conversion : ArithShift  BitShiftNumber=-6
  Measured Iab PU : Outport
  wires:
  Q17 per unit conversion/1 -> Data Type Conversion/1
  Data Type Conversion1/1 -> Measured Iab PU/1
  In/1 -> Q17 per unit conversion/1
  Data Type Conversion/1 -> Data Type Conversion1/1

== system model/Current Controller/Control Variant Subsystem/PI Controller/Phase Current Calculator/Variant Subsystem1/Float ==
  In : Inport
  Current Sense Gain : Gain  Gain=PU_System.I_base/1.65  RndMeth=Simplest  OutDataTypeStr=Inherit: Same as input
  Get_ADC_Volt : Gain  Gain=1.65/2048  OutDataTypeStr=dataType  RndMeth=Simplest
  PU_Conversion : Gain  Gain=1/PU_System.I_base  RndMeth=Simplest  OutDataTypeStr=Inherit: Same as input
  Measured Iab PU : Outport
  wires:
  Current Sense Gain/1 -> PU_Conversion/1
  In/1 -> Get_ADC_Volt/1
  Get_ADC_Volt/1 -> Current Sense Gain/1
  PU_Conversion/1 -> Measured Iab PU/1

== system model/Current Controller/Control Variant Subsystem/TD3 Agent/Phase Current Calculator/Variant Subsystem1/Fixed Point ==
  In : Inport
  Data Type Conversion : DataTypeConversion  OutDataTypeStr=fixdt(1,32,17)  ConvertRealWorld=Stored Integer (SI)  RndMeth=Simplest
  Data Type Conversion1 : DataTypeConversion  OutDataTypeStr=dataType  RndMeth=Simplest
  Q17 per unit conversion : ArithShift  BitShiftNumber=-6
  Measured Iab PU : Outport
  wires:
  Q17 per unit conversion/1 -> Data Type Conversion/1
  Data Type Conversion1/1 -> Measured Iab PU/1
  In/1 -> Q17 per unit conversion/1
  Data Type Conversion/1 -> Data Type Conversion1/1

== system model/Current Controller/Control Variant Subsystem/TD3 Agent/Phase Current Calculator/Variant Subsystem1/Float ==
  In : Inport
  Current Sense Gain : Gain  Gain=PU_System.I_base/1.65  RndMeth=Simplest  OutDataTypeStr=Inherit: Same as input
  Get_ADC_Volt : Gain  Gain=1.65/2048  OutDataTypeStr=dataType  RndMeth=Simplest
  PU_Conversion : Gain  Gain=1/PU_System.I_base  RndMeth=Simplest  OutDataTypeStr=Inherit: Same as input
  Measured Iab PU : Outport
  wires:
  Current Sense Gain/1 -> PU_Conversion/1
  In/1 -> Get_ADC_Volt/1
  Get_ADC_Volt/1 -> Current Sense Gain/1
  PU_Conversion/1 -> Measured Iab PU/1
